simulink subsystem "DCDriver_PWM"  (R2025a)
settings: Solver=VariableStepAuto  StartTime=0.0  StopTime=10.0  RelTol=1e-3
model mask{PWM_rate=0, Supply_Vcc=0}
  mask prompts: PWM_rate "PWM Frequency (Hz)"; Supply_Vcc "Supply Voltage (V)"
libraries: fl_lib x6, ee_lib x2, nesl_utility x2, simulink x1
settings Model: DataDictionary=neck_mk3.sldd  EnableAccessToBaseWorkspace=off  DefaultTestHarness=DCDriver_PWM_Harness1  Creator=upattacini  LastModifiedBy=upattacini
settings RTWCC: GPUComputeCapability=3.5

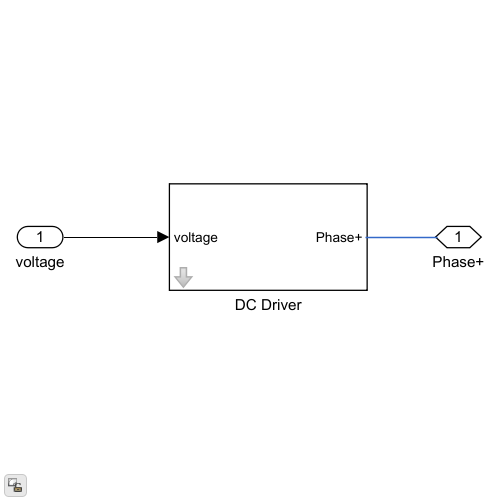
[thumbnail: Simulink's stored preview of the top-level diagram]
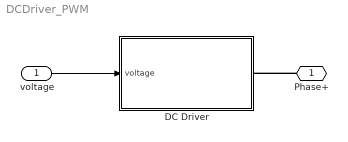
== system DCDriver_PWM ==
  voltage : Inport  Unit=%  PortDimensions=1
  DC Driver : Subsystem  mask{PWM_rate=PWM_rate, Supply_Vcc=Supply_Vcc}
      mask prompts: PWM_rate "PWM Frequency (Hz)"; Supply_Vcc "Supply Voltage (V)"
  Phase+ : PMIOPort  Side=Right
  wires:
  voltage/1 -> DC Driver/1(voltage)
  connections:
  Phase+/RConn1 -- DC Driver/RConn1

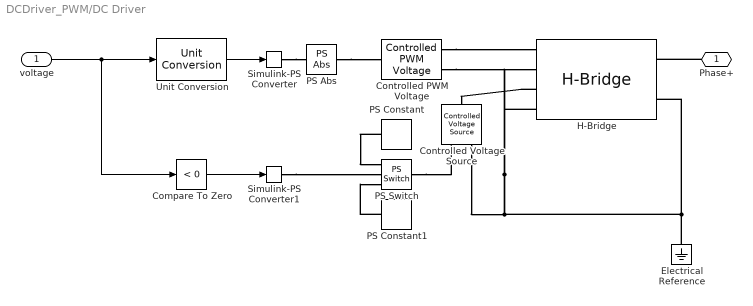
== system DCDriver_PWM/DC Driver ==
  voltage : Inport
  Compare To Zero : simulink/Logic and Bit Operations/Compare To Zero  relop=<  OutDataTypeStr=uint8
  Controlled PWM Voltage : ee_lib/Integrated Circuits/Controlled PWM Voltage  F=PWM_rate kHz  TD=0 s  pulse_width_offset=0 s  pulse_min=0 s  pwm_or_av=ee.enum.pwm_or_av.averaged  event_type=ee.enum.ic.event.asynchronous  sample_time=1e-6 s  Vmin=0 V  Vmax=24 V  Vm=Supply_Vcc V  u_min=0  u_max=1
      settings: InternalSimscapePortConfiguration="{\"Bottom\":[],\"Left\":[{\"id\":\"u\",\"label\":\"u\",\"type\":\"input\"}],\"Right\":[{\"id\":\"p2\",\"label\":\"PWM\",\"type\":\"foundation.electrical.electrical\"},{\"id\":\"n2\",\"label\":\"REF\",\"type\":\"foundation.electrical.electrical\"}],\"Top\":[]}"
  Controlled Voltage Source : fl_lib/Electrical/Electrical Sources/Controlled Voltage Source
  Electrical Reference : fl_lib/Electrical/Electrical Elements/Electrical Reference
  H-Bridge : ee_lib/Semiconductors & Converters/Converters/H-Bridge  supply_ports=ee.enum.supply_ports.hidesupply  pwm_or_av=ee.enum.pwm_or_av.averaged  regenerative_braking_mode=ee.enum.converters.regenerative_braking_mode.always_enabled  discontinuous=ee.enum.current_profile.continuous  freewheeling_mode=ee.enum.converters.freewheeling_mode.one_switch_one_diode  Rload=10 Ohm  Lload=1e-5 H  F=10 kHz  Venable=2.5 V  Vmax=Supply_Vcc V  Vreverse=2.5 V  Vbrake=2.5 V  Vm=Supply_Vcc V  Ron=0.1 Ohm  Don=0.05 Ohm  Goff=1e-6 S  Tmeas=298.15 K  Ron2=0.1 Ohm  Don2=0.05 Ohm  Tmeas2=398.15 K  thermal_mass=100 J/K  initial_temperature=298.15 K
  PS Abs : fl_lib/Physical Signals/Nonlinear Operators/PS Abs  ZeroCross=true
      settings: InternalSimscapePortConfiguration="{\"Bottom\":[],\"Left\":[{\"id\":\"I\",\"label\":\"\",\"type\":\"input\"}],\"Right\":[{\"id\":\"O\",\"label\":\"\",\"type\":\"output\"}],\"Top\":[]}"
  PS Constant : fl_lib/Physical Signals/Sources/PS Constant  constant=5 V
  PS Constant1 : fl_lib/Physical Signals/Sources/PS Constant  constant=0 V
  PS Switch : fl_lib/Physical Signals/Nonlinear Operators/PS Switch  Threshold=0.5  ZeroCross=true
      settings: InternalSimscapePortConfiguration="{\"Bottom\":[],\"Left\":[{\"id\":\"I1\",\"label\":\"\",\"type\":\"input\"},{\"id\":\"I2\",\"label\":\"\",\"type\":\"input\"},{\"id\":\"I3\",\"label\":\"\",\"type\":\"input\"}],\"Right\":[{\"id\":\"O\",\"label\":\"\",\"type\":\"output\"}],\"Top\":[]}"
  Simulink-PS Converter : nesl_utility/Simulink-PS Converter  PhysicalDomain=network_engine_domain  SubClassName=ps_input  LeftPortType=input  RightPortType=output  PseudoPeriodic=off  Frequencies=[]  NoiseDistribution=none  NoiseParameters=[]  Unit=1  AffineConversion=off  FilteringAndDerivatives=provide  SimscapeFilterOrder=1  InputFilterTimeConstant=0.001  UdotUserProvided=0
  Simulink-PS Converter1 : nesl_utility/Simulink-PS Converter  PhysicalDomain=network_engine_domain  SubClassName=ps_input  LeftPortType=input  RightPortType=output  PseudoPeriodic=off  Frequencies=[]  NoiseDistribution=none  NoiseParameters=[]  Unit=1  AffineConversion=off  FilteringAndDerivatives=provide  SimscapeFilterOrder=1  InputFilterTimeConstant=0.001  UdotUserProvided=0
  Unit Conversion : UnitConversion
  Phase+ : PMIOPort  Side=Right
  wires:
  Compare To Zero/1 -> Simulink-PS Converter1/1
  Unit Conversion/1 -> Simulink-PS Converter/1
  voltage/1 -> Compare To Zero/1, Unit Conversion/1
  connections:
  PS Constant1/RConn1 -- PS Switch/LConn3
  H-Bridge/LConn3 -- Controlled Voltage Source/LConn1
  PS Constant/RConn1 -- PS Switch/LConn1
  Simulink-PS Converter/RConn1 -- PS Abs/LConn1
  PS Switch/RConn1 -- Controlled Voltage Source/RConn1
  Simulink-PS Converter1/RConn1 -- PS Switch/LConn2
  Controlled PWM Voltage/RConn1 -- H-Bridge/LConn1
  PS Abs/RConn1 -- Controlled PWM Voltage/LConn1
  Phase+/RConn1 -- H-Bridge/RConn1
  Electrical Reference/LConn1 -- H-Bridge/RConn2 -- H-Bridge/LConn4 -- H-Bridge/LConn2 -- Controlled PWM Voltage/RConn2 -- Controlled Voltage Source/RConn2
